simulink model "CLA_Sample"  (R2022b)
settings: Solver=FixedStepAuto  StartTime=0.0  StopTime=Inf  RelTol=1e-3  EnableMultiTasking=on
model workspace (MAT data in the model file):
  ADC_Gain = 1241.21212121
  DAC_Gain = 0.000805860805861
  Inductor_Current_Divider_Gain_Phase_A = 33.4
  Inductor_Current_Divider_Gain_Phase_B = 33.4
  Vbulk_Divider_Gain = 276.854928018
  Vin_Divider_Gain = 556.17352614
undefined symbols (not defined in the file or in its folder): GPTRIP1SEL, GPTRIP2SEL, SCI_A_Transmit, SCI_A_Transmit_Current_Suffix, SCI_A_Transmit_one_shot_Suffix, SCI_A_Transmit_Polarity_Suffix, SCI_A_Transmit_relay_Suffix, SCI_A_Transmit_Vbulk_Suffix, SCI_A_Transmit_Vin_rms_Suffix, SCI_A_Transmit_Vin_Suffix, SCI_A_Transmit_Vmid_Suffix, SCI_A_Transmit_Vp_Suffix, SCI_A_Transmit_Vpfc_Suffix, TZ1, TZ2
libraries: c280xlib x33, simulink x17, c2802xlib x15, c2000lib x1, c2806xlib x1
(part 3 of 5)

== system CLA_Sample/Calibration,RMS, Fault Protection @5kHz/Fault checking/If Action Subsystem ==
  note: Do other fault checks here.
  note: O/P Bulk_UVP-> working but still not perfect.
      | Add more conditons during start up(Not to trigger)
  Action Port : ActionPort  ActionPortLabel=if(u1 ==1)
  Fault Check (Bulk UVP) : Subsystem  Commented=on  TreatAsAtomicUnit=on
  Function-Call Generator : simulink/Ports & Subsystems/Function-Call Generator  sample_time=-1  numberOfIterations=1  DisallowWideOutput=off
  Function-Call Split : FunctionCallSplit  IconShape=distinctive  NumOutputPorts=9  OutputPortLayout=default
  Output Voltage_Latch_OVP : Subsystem  TreatAsAtomicUnit=on
  PFC_en_update_3Phase : Subsystem  TreatAsAtomicUnit=on
  PFC_en_update_Phase_A : Subsystem  TreatAsAtomicUnit=on
  PFC_en_update_Phase_B : Subsystem  TreatAsAtomicUnit=on
  PFC_en_update_Phase_C : Subsystem  TreatAsAtomicUnit=on
  Phase_A_Fault : Subsystem  TreatAsAtomicUnit=on
  Phase_B_Fault : Subsystem  TreatAsAtomicUnit=on
  Phase_C_Fault : Subsystem  TreatAsAtomicUnit=on
  wires:
  Function-Call Generator/1 -> Function-Call Split/1
  Function-Call Split/1 -> Fault Check (Bulk UVP)/Trigger
  Function-Call Split/2 -> Output Voltage_Latch_OVP/Trigger
  Function-Call Split/3 -> Phase_A_Fault/Trigger
  Function-Call Split/4 -> Phase_B_Fault/Trigger
  Function-Call Split/5 -> Phase_C_Fault/Trigger
  Function-Call Split/6 -> PFC_en_update_Phase_A/Trigger
  Function-Call Split/7 -> PFC_en_update_Phase_B/Trigger
  Function-Call Split/8 -> PFC_en_update_Phase_C/Trigger
  Function-Call Split/9 -> PFC_en_update_3Phase/Trigger

== system CLA_Sample/Calibration,RMS, Fault Protection @5kHz/Polarity & Near Zero check/Polarity_Near_zero_Phase_A ==
  note: Unit in Volt
  function : TriggerPort  TriggerType=function-call  VariantControl=(inherit)
  Chart : Stateflow chart  TreatAsAtomicUnit=on
  Constant7 : Constant  Value=0
  Data Store Read2 : DataStoreRead  DataStoreName=Vin_ADC_Average_Phase_A  IndexOptions=Index vector (dialog)  Indices=1  OutputSizes=1
  Data Store Read5 : DataStoreRead  DataStoreName=Vin_1_65_ADC_Phase_A  IndexOptions=Index vector (dialog)  Indices=1  OutputSizes=1
  Data Store Write1 : DataStoreWrite  DataStoreName=Near_Zero_Bar_Phase_A  IndexOptions=Index vector (dialog)  Indices=1  OutputSizes=1
  Data Store Write3 : DataStoreWrite  DataStoreName=Polarity_Phase_A  IndexOptions=Index vector (dialog)  Indices=1  OutputSizes=1
  Near Zero_7V_Analog : Constant  Value=7
  Near_zero : c280xlib/Digital Output  Commented=on  GPIO_Number=GPIO16~GPIO23  GPIO_Bit0=off  GPIO_BIT0_Toggle=off  GPIO_Bit1=off  GPIO_BIT1_Toggle=off  GPIO_Bit2=off  GPIO_BIT2_Toggle=off  GPIO_Bit3=off  GPIO_BIT3_Toggle=off  GPIO_Bit4=off  GPIO_BIT4_Toggle=off  GPIO_Bit5=off  GPIO_BIT5_Toggle=off  GPIO_Bit6=on  GPIO_BIT6_Toggle=off  GPIO_Bit7=off  GPIO_BIT7_Toggle=off
  Polarity : c280xlib/Digital Output  Commented=on  GPIO_Number=GPIO24~GPIO31  GPIO_Bit0=off  GPIO_BIT0_Toggle=off  GPIO_Bit1=on  GPIO_BIT1_Toggle=off  GPIO_Bit2=off  GPIO_BIT2_Toggle=off  GPIO_Bit3=off  GPIO_BIT3_Toggle=off  GPIO_Bit4=off  GPIO_BIT4_Toggle=off  GPIO_Bit5=off  GPIO_BIT5_Toggle=off  GPIO_Bit6=off  GPIO_BIT6_Toggle=off  GPIO_Bit7=off  GPIO_BIT7_Toggle=off
  Subtract2 : Sum  Inputs=+-
  Volt to Number : Subsystem
  wires:
  Constant7/1 -> Chart/2(Vref)
  Volt to Number/1(Out1) -> Chart/3(VZCD_Gap)
  Chart/2(Near_zero) -> Near_zero/1, Data Store Write1/1
  Near Zero_7V_Analog/1 -> Volt to Number/1(In1)
  Chart/1(Polarity) -> Polarity/1, Data Store Write3/1
  Data Store Read5/1 -> Subtract2/2
  Data Store Read2/1 -> Subtract2/1
  Subtract2/1 -> Chart/1(input)

== system CLA_Sample/Calibration,RMS, Fault Protection @5kHz/Polarity & Near Zero check/Polarity_Near_zero_Phase_B ==
  note: Unit in Volt
  function : TriggerPort  TriggerType=function-call  VariantControl=(inherit)
  Chart : Stateflow chart  TreatAsAtomicUnit=on
  Constant7 : Constant  Value=0
  Data Store Read2 : DataStoreRead  DataStoreName=Vin_ADC_Average_Phase_B  IndexOptions=Index vector (dialog)  Indices=1  OutputSizes=1
  Data Store Read5 : DataStoreRead  DataStoreName=Vin_1_65_ADC_Phase_B  IndexOptions=Index vector (dialog)  Indices=1  OutputSizes=1
  Data Store Write1 : DataStoreWrite  DataStoreName=Near_Zero_Bar_Phase_B  IndexOptions=Index vector (dialog)  Indices=1  OutputSizes=1
  Data Store Write3 : DataStoreWrite  DataStoreName=Polarity_Phase_B  IndexOptions=Index vector (dialog)  Indices=1  OutputSizes=1
  Near Zero_7V_Analog : Constant  Value=7
  Near_zero : c280xlib/Digital Output  Commented=on  GPIO_Number=GPIO16~GPIO23  GPIO_Bit0=off  GPIO_BIT0_Toggle=off  GPIO_Bit1=off  GPIO_BIT1_Toggle=off  GPIO_Bit2=off  GPIO_BIT2_Toggle=off  GPIO_Bit3=off  GPIO_BIT3_Toggle=off  GPIO_Bit4=off  GPIO_BIT4_Toggle=off  GPIO_Bit5=off  GPIO_BIT5_Toggle=off  GPIO_Bit6=on  GPIO_BIT6_Toggle=off  GPIO_Bit7=off  GPIO_BIT7_Toggle=off
  Polarity : c280xlib/Digital Output  Commented=on  GPIO_Number=GPIO24~GPIO31  GPIO_Bit0=off  GPIO_BIT0_Toggle=off  GPIO_Bit1=on  GPIO_BIT1_Toggle=off  GPIO_Bit2=off  GPIO_BIT2_Toggle=off  GPIO_Bit3=off  GPIO_BIT3_Toggle=off  GPIO_Bit4=off  GPIO_BIT4_Toggle=off  GPIO_Bit5=off  GPIO_BIT5_Toggle=off  GPIO_Bit6=off  GPIO_BIT6_Toggle=off  GPIO_Bit7=off  GPIO_BIT7_Toggle=off
  Subtract2 : Sum  Inputs=+-
  Volt to Number : Subsystem
  wires:
  Constant7/1 -> Chart/2(Vref)
  Volt to Number/1(Out1) -> Chart/3(VZCD_Gap)
  Chart/2(Near_zero) -> Near_zero/1, Data Store Write1/1
  Near Zero_7V_Analog/1 -> Volt to Number/1(In1)
  Chart/1(Polarity) -> Polarity/1, Data Store Write3/1
  Data Store Read5/1 -> Subtract2/2
  Data Store Read2/1 -> Subtract2/1
  Subtract2/1 -> Chart/1(input)

== system CLA_Sample/Calibration,RMS, Fault Protection @5kHz/Polarity & Near Zero check/Polarity_Near_zero_Phase_C ==
  note: Unit in Volt
  function : TriggerPort  TriggerType=function-call  VariantControl=(inherit)
  Chart : Stateflow chart  TreatAsAtomicUnit=on
  Constant7 : Constant  Value=0
  Data Store Read2 : DataStoreRead  DataStoreName=Vin_ADC_Average_Phase_C  IndexOptions=Index vector (dialog)  Indices=1  OutputSizes=1
  Data Store Read5 : DataStoreRead  DataStoreName=Vin_1_65_ADC_Phase_C  IndexOptions=Index vector (dialog)  Indices=1  OutputSizes=1
  Data Store Write1 : DataStoreWrite  DataStoreName=Near_Zero_Bar_Phase_C  IndexOptions=Index vector (dialog)  Indices=1  OutputSizes=1
  Data Store Write3 : DataStoreWrite  DataStoreName=Polarity_Phase_C  IndexOptions=Index vector (dialog)  Indices=1  OutputSizes=1
  Near Zero_7V_Analog : Constant  Value=7
  Near_zero : c280xlib/Digital Output  Commented=on  GPIO_Number=GPIO16~GPIO23  GPIO_Bit0=off  GPIO_BIT0_Toggle=off  GPIO_Bit1=off  GPIO_BIT1_Toggle=off  GPIO_Bit2=off  GPIO_BIT2_Toggle=off  GPIO_Bit3=off  GPIO_BIT3_Toggle=off  GPIO_Bit4=off  GPIO_BIT4_Toggle=off  GPIO_Bit5=off  GPIO_BIT5_Toggle=off  GPIO_Bit6=on  GPIO_BIT6_Toggle=off  GPIO_Bit7=off  GPIO_BIT7_Toggle=off
  Polarity : c280xlib/Digital Output  Commented=on  GPIO_Number=GPIO24~GPIO31  GPIO_Bit0=off  GPIO_BIT0_Toggle=off  GPIO_Bit1=on  GPIO_BIT1_Toggle=off  GPIO_Bit2=off  GPIO_BIT2_Toggle=off  GPIO_Bit3=off  GPIO_BIT3_Toggle=off  GPIO_Bit4=off  GPIO_BIT4_Toggle=off  GPIO_Bit5=off  GPIO_BIT5_Toggle=off  GPIO_Bit6=off  GPIO_BIT6_Toggle=off  GPIO_Bit7=off  GPIO_BIT7_Toggle=off
  Subtract2 : Sum  Inputs=+-
  Volt to Number : Subsystem
  wires:
  Constant7/1 -> Chart/2(Vref)
  Volt to Number/1(Out1) -> Chart/3(VZCD_Gap)
  Chart/2(Near_zero) -> Near_zero/1, Data Store Write1/1
  Near Zero_7V_Analog/1 -> Volt to Number/1(In1)
  Chart/1(Polarity) -> Polarity/1, Data Store Write3/1
  Data Store Read5/1 -> Subtract2/2
  Data Store Read2/1 -> Subtract2/1
  Subtract2/1 -> Chart/1(input)

== system CLA_Sample/Calibration,RMS, Fault Protection @5kHz/Relay control/ADC Gain ==
  In1 : Inport
  Gain : Gain  Gain=ADC_Gain
  Gain1 : Gain  Gain=1/Vin_Divider_Gain
  Out1 : Outport
  wires:
  Gain1/1 -> Gain/1
  In1/1 -> Gain1/1
  Gain/1 -> Out1/1

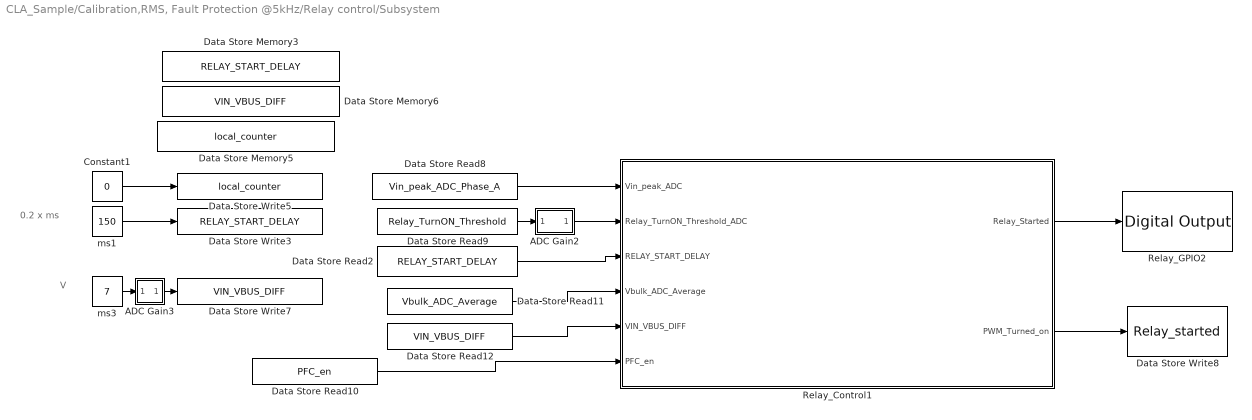
== system CLA_Sample/Calibration,RMS, Fault Protection @5kHz/Relay control/Subsystem ==
  note: 0.2 x ms
  note: V
  ADC Gain2 : Subsystem
  ADC Gain3 : Subsystem
  Constant1 : Constant  Value=0
  Data Store Memory3 : DataStoreMemory  DataStoreName=RELAY_START_DELAY  WriteAfterWriteMsg=warning  ShowAdditionalParam=off
  Data Store Memory5 : DataStoreMemory  DataStoreName=local_counter  WriteAfterWriteMsg=warning  ShowAdditionalParam=off
  Data Store Memory6 : DataStoreMemory  DataStoreName=VIN_VBUS_DIFF  WriteAfterWriteMsg=warning  ShowAdditionalParam=off
  Data Store Read10 : DataStoreRead  DataStoreName=PFC_en  IndexOptions=Index vector (dialog)  Indices=1  OutputSizes=1
  Data Store Read11 : DataStoreRead  DataStoreName=Vbulk_ADC_Average  IndexOptions=Index vector (dialog)  Indices=1  OutputSizes=1
  Data Store Read12 : DataStoreRead  DataStoreName=VIN_VBUS_DIFF  IndexOptions=Index vector (dialog)  Indices=1  OutputSizes=1
  Data Store Read2 : DataStoreRead  DataStoreName=RELAY_START_DELAY  IndexOptions=Index vector (dialog)  Indices=1  OutputSizes=1
  Data Store Read8 : DataStoreRead  DataStoreName=Vin_peak_ADC_Phase_A  IndexOptions=Index vector (dialog)  Indices=1  OutputSizes=1
  Data Store Read9 : DataStoreRead  DataStoreName=Relay_TurnON_Threshold  IndexOptions=Index vector (dialog)  Indices=1  OutputSizes=1
  Data Store Write3 : DataStoreWrite  DataStoreName=RELAY_START_DELAY  IndexOptions=Index vector (dialog)  Indices=1  OutputSizes=1
  Data Store Write5 : DataStoreWrite  DataStoreName=local_counter  IndexOptions=Index vector (dialog)  Indices=1  OutputSizes=1
  Data Store Write7 : DataStoreWrite  DataStoreName=VIN_VBUS_DIFF  IndexOptions=Index vector (dialog)  Indices=1  OutputSizes=1
  Data Store Write8 : DataStoreWrite  DataStoreName=Relay_started  IndexOptions=Index vector (dialog)  Indices=1  OutputSizes=1
  Relay_Control1 : Stateflow chart  TreatAsAtomicUnit=on
  Relay_GPIO2 : c280xlib/Digital Output  GPIO_Number=GPIO8~GPIO15  GPIO_Bit0=on  GPIO_BIT0_Toggle=off  GPIO_Bit1=off  GPIO_BIT1_Toggle=off  GPIO_Bit2=off  GPIO_BIT2_Toggle=off  GPIO_Bit3=off  GPIO_BIT3_Toggle=off  GPIO_Bit4=off  GPIO_BIT4_Toggle=off  GPIO_Bit5=off  GPIO_BIT5_Toggle=off  GPIO_Bit6=off  GPIO_BIT6_Toggle=off  GPIO_Bit7=off  GPIO_BIT7_Toggle=off
  ms1 : Constant  Value=150
  ms3 : Constant  Value=7
  wires:
  Data Store Read8/1 -> Relay_Control1/1(Vin_peak_ADC)
  Data Store Read11/1 -> Relay_Control1/4(Vbulk_ADC_Average)
  Relay_Control1/2(PWM_Turned_on) -> Data Store Write8/1
  Data Store Read9/1 -> ADC Gain2/1(In1)
  Data Store Read2/1 -> Relay_Control1/3(RELAY_START_DELAY)
  Data Store Read10/1 -> Relay_Control1/6(PFC_en)
  ADC Gain3/1(Out1) -> Data Store Write7/1
  ms1/1 -> Data Store Write3/1
  ms3/1 -> ADC Gain3/1(In1)
  Relay_Control1/1(Relay_Started) -> Relay_GPIO2/1
  ADC Gain2/1(Out1) -> Relay_Control1/2(Relay_TurnON_Threshold_ADC)
  Constant1/1 -> Data Store Write5/1
  Data Store Read12/1 -> Relay_Control1/5(VIN_VBUS_DIFF)

== system CLA_Sample/Calibration,RMS, Fault Protection @5kHz/Voltage RMS//Averag Calculation/Phase_A ==
  function : TriggerPort  TriggerType=function-call  VariantControl=(inherit)
  Function-Call Generator : simulink/Ports & Subsystems/Function-Call Generator  sample_time=-1  numberOfIterations=1  DisallowWideOutput=off
  Function-Call Split : FunctionCallSplit  IconShape=distinctive  NumOutputPorts=3  OutputPortLayout=default
  RMS Current Calculation_Phase_A : Subsystem  TreatAsAtomicUnit=on
  RMS Voltage Calculation_Phase_A : Subsystem  TreatAsAtomicUnit=on
  Vin_ADC Averaging_Phase_A : Subsystem  TreatAsAtomicUnit=on
  wires:
  Function-Call Generator/1 -> Function-Call Split/1
  Function-Call Split/1 -> RMS Voltage Calculation_Phase_A/Trigger
  Function-Call Split/2 -> RMS Current Calculation_Phase_A/Trigger
  Function-Call Split/3 -> Vin_ADC Averaging_Phase_A/Trigger

== system CLA_Sample/Calibration,RMS, Fault Protection @5kHz/Voltage RMS//Averag Calculation/Phase_B ==
  function : TriggerPort  TriggerType=function-call  VariantControl=(inherit)
  Function-Call Generator : simulink/Ports & Subsystems/Function-Call Generator  sample_time=-1  numberOfIterations=1  DisallowWideOutput=off
  Function-Call Split : FunctionCallSplit  IconShape=distinctive  NumOutputPorts=3  OutputPortLayout=default
  RMS Current Calculation_Phase_B : Subsystem  TreatAsAtomicUnit=on
  RMS Voltage Calculation_Phase_B : Subsystem  TreatAsAtomicUnit=on
  Vin_ADC Averaging_Phase_B : Subsystem  TreatAsAtomicUnit=on
  wires:
  Function-Call Generator/1 -> Function-Call Split/1
  Function-Call Split/1 -> RMS Voltage Calculation_Phase_B/Trigger
  Function-Call Split/2 -> RMS Current Calculation_Phase_B/Trigger
  Function-Call Split/3 -> Vin_ADC Averaging_Phase_B/Trigger

== system CLA_Sample/Calibration,RMS, Fault Protection @5kHz/Voltage RMS//Averag Calculation/Phase_C ==
  function : TriggerPort  TriggerType=function-call  VariantControl=(inherit)
  Function-Call Generator : simulink/Ports & Subsystems/Function-Call Generator  sample_time=-1  numberOfIterations=1  DisallowWideOutput=off
  Function-Call Split : FunctionCallSplit  IconShape=distinctive  NumOutputPorts=3  OutputPortLayout=default
  RMS Current Calculation_Phase_C : Subsystem  TreatAsAtomicUnit=on
  RMS Voltage Calculation_Phase_C : Subsystem  TreatAsAtomicUnit=on
  Vin_ADC Averaging_Phase_C : Subsystem  TreatAsAtomicUnit=on
  wires:
  Function-Call Generator/1 -> Function-Call Split/1
  Function-Call Split/1 -> RMS Voltage Calculation_Phase_C/Trigger
  Function-Call Split/2 -> RMS Current Calculation_Phase_C/Trigger
  Function-Call Split/3 -> Vin_ADC Averaging_Phase_C/Trigger

== system CLA_Sample/Calibration,RMS, Fault Protection @5kHz/Voltage RMS//Averag Calculation/Vbulk_ADC Averaging ==
  note: Low pass filter :
      | 1kHz bandwidth with 5kHz switching freq
  function : TriggerPort  TriggerType=function-call  VariantControl=(inherit)
  Chart1 : Stateflow chart  TreatAsAtomicUnit=on
  Constant1 : Constant  Value=0.38586954
  Constant2 : Constant  Value=0.38586954
  Constant3 : Constant  Value=-0.22826091
  Data Store Read1 : DataStoreRead  DataStoreName=Vbulk_ADC  IndexOptions=Index vector (dialog)  Indices=1  OutputSizes=1
  Vout_ADC_Average : DataStoreWrite  DataStoreName=Vbulk_ADC_Average  IndexOptions=Index vector (dialog)  Indices=1  OutputSizes=1
  wires:
  Chart1/1(output_y) -> Vout_ADC_Average/1
  Data Store Read1/1 -> Chart1/1(input_u)
  [b0] -> Chart1/2(b0)
  [b1] -> Chart1/3(b1)
  [a1] -> Chart1/4(a1)
  Constant2/1 -> [b1]
  Constant1/1 -> [b0]
  Constant3/1 -> [a1]

== system CLA_Sample/PWM Update @65KHz/Closed loop PWM generation (Control)/If Action Subsystem ==
  Action Port : ActionPort  ActionPortLabel=if((u1 ==1) & (u2==1))
  CLA Task : c2806xlib/CLA Task  taskNumber=1  intSource=Software  wait=off  sampleTime=0.2  claType=0  softTrigSelected=1  enableInterrupt=on
  Function-Call Subsystem : Subsystem  TreatAsAtomicUnit=on
  wires:
  CLA Task/1 -> Function-Call Subsystem/Trigger

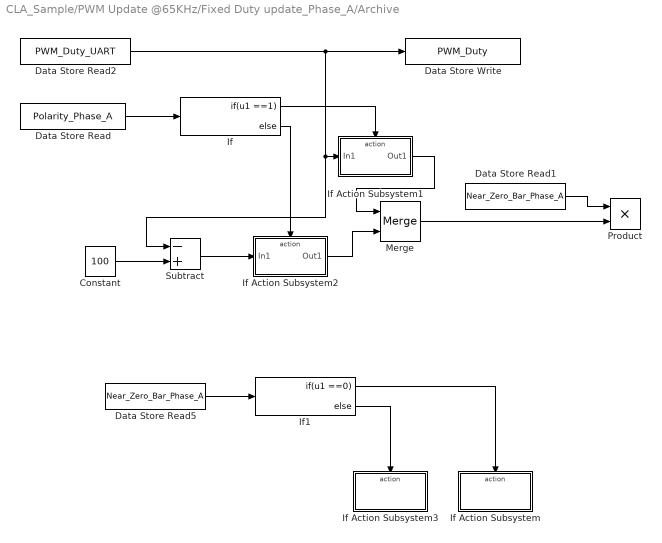
== system CLA_Sample/PWM Update @65KHz/Fixed Duty update_Phase_A/Archive ==
  Constant : Constant  Value=100
  Data Store Read : DataStoreRead  DataStoreName=Polarity_Phase_A  IndexOptions=Index vector (dialog)  Indices=1  OutputSizes=1
  Data Store Read1 : DataStoreRead  DataStoreName=Near_Zero_Bar_Phase_A  IndexOptions=Index vector (dialog)  Indices=1  OutputSizes=1
  Data Store Read2 : DataStoreRead  DataStoreName=PWM_Duty_UART  IndexOptions=Index vector (dialog)  Indices=1  OutputSizes=1
  Data Store Read5 : DataStoreRead  DataStoreName=Near_Zero_Bar_Phase_A  IndexOptions=Index vector (dialog)  Indices=1  OutputSizes=1
  Data Store Write : DataStoreWrite  DataStoreName=PWM_Duty  IndexOptions=Index vector (dialog)  Indices=1  OutputSizes=1
  If : If  IfExpression=u1 ==1
  If Action Subsystem : Subsystem  TreatAsAtomicUnit=on
  If Action Subsystem1 : Subsystem  TreatAsAtomicUnit=on
  If Action Subsystem2 : Subsystem  TreatAsAtomicUnit=on
  If Action Subsystem3 : Subsystem  TreatAsAtomicUnit=on
  If1 : If  IfExpression=u1 ==0
  Merge : Merge
  Product : Product
  Subtract : Sum  Inputs=-+
  wires:
  If/1 -> If Action Subsystem1/Action
  Data Store Read2/1 -> If Action Subsystem1/1(In1), Subtract/1, Data Store Write/1
  Merge/1 -> Product/2
  If Action Subsystem2/1(Out1) -> Merge/2
  Constant/1 -> Subtract/2
  Data Store Read/1 -> If/1
  Subtract/1 -> If Action Subsystem2/1(In1)
  Data Store Read1/1 -> Product/1
  If/2 -> If Action Subsystem2/Action
  If Action Subsystem1/1(Out1) -> Merge/1
  If1/1 -> If Action Subsystem/Action
  Data Store Read5/1 -> If1/1
  If1/2 -> If Action Subsystem3/Action

== system CLA_Sample/PWM Update @65KHz/Fixed Duty update_Phase_A/If Action Subsystem3 ==
  Action Port : ActionPort  ActionPortLabel=if(u1==1 & u2==0)
  Constant : Constant
  Digital Output : c280xlib/Digital Output  GPIO_Number=GPIO16~GPIO23  GPIO_Bit0=off  GPIO_BIT0_Toggle=off  GPIO_Bit1=off  GPIO_BIT1_Toggle=off  GPIO_Bit2=off  GPIO_BIT2_Toggle=off  GPIO_Bit3=off  GPIO_BIT3_Toggle=off  GPIO_Bit4=off  GPIO_BIT4_Toggle=off  GPIO_Bit5=off  GPIO_BIT5_Toggle=off  GPIO_Bit6=on  GPIO_BIT6_Toggle=off  GPIO_Bit7=off  GPIO_BIT7_Toggle=off
  wires:
  Constant/1 -> Digital Output/1

== system CLA_Sample/PWM Update @65KHz/Fixed Duty update_Phase_A/If Action Subsystem4 ==
  Action Port : ActionPort  ActionPortLabel=elseif(u1==1 & u2==1)
  Constant : Constant  Value=0
  Digital Output : c280xlib/Digital Output  GPIO_Number=GPIO16~GPIO23  GPIO_Bit0=off  GPIO_BIT0_Toggle=off  GPIO_Bit1=off  GPIO_BIT1_Toggle=off  GPIO_Bit2=off  GPIO_BIT2_Toggle=off  GPIO_Bit3=off  GPIO_BIT3_Toggle=off  GPIO_Bit4=off  GPIO_BIT4_Toggle=off  GPIO_Bit5=off  GPIO_BIT5_Toggle=off  GPIO_Bit6=on  GPIO_BIT6_Toggle=off  GPIO_Bit7=off  GPIO_BIT7_Toggle=off
  wires:
  Constant/1 -> Digital Output/1

== system CLA_Sample/PWM Update @65KHz/Fixed Duty update_Phase_A/Subsystem1 ==
  Frequency(kHz) : Inport
  Duty(%) : Inport  Port=2
  Constant1 : Constant  Value=90E6
  Divide : Product  Inputs=*/  RndMeth=Zero  SaturateOnIntegerOverflow=on
  Gain : Gain  Gain=1000
  Gain1 : Gain  Gain=1/100
  Gain2 : Gain  Gain=0.5
  Product1 : Product
  Out1 : Outport
  Out2 : Outport  Port=2
  Out3 : Outport  Port=3
  wires:
  Gain2/1 -> Out3/1
  Gain1/1 -> Product1/2
  Product1/1 -> Gain2/1, Out2/1
  Duty(%)/1 -> Gain1/1
  Divide/1 -> Out1/1, Product1/1
  Gain/1 -> Divide/2
  Constant1/1 -> Divide/1
  Frequency(kHz)/1 -> Gain/1

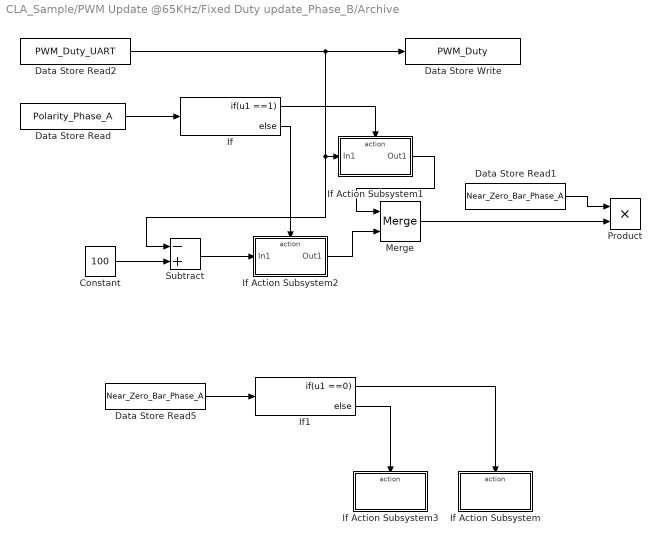
== system CLA_Sample/PWM Update @65KHz/Fixed Duty update_Phase_B/Archive ==
  Constant : Constant  Value=100
  Data Store Read : DataStoreRead  DataStoreName=Polarity_Phase_A  IndexOptions=Index vector (dialog)  Indices=1  OutputSizes=1
  Data Store Read1 : DataStoreRead  DataStoreName=Near_Zero_Bar_Phase_A  IndexOptions=Index vector (dialog)  Indices=1  OutputSizes=1
  Data Store Read2 : DataStoreRead  DataStoreName=PWM_Duty_UART  IndexOptions=Index vector (dialog)  Indices=1  OutputSizes=1
  Data Store Read5 : DataStoreRead  DataStoreName=Near_Zero_Bar_Phase_A  IndexOptions=Index vector (dialog)  Indices=1  OutputSizes=1
  Data Store Write : DataStoreWrite  DataStoreName=PWM_Duty  IndexOptions=Index vector (dialog)  Indices=1  OutputSizes=1
  If : If  IfExpression=u1 ==1
  If Action Subsystem : Subsystem  TreatAsAtomicUnit=on
  If Action Subsystem1 : Subsystem  TreatAsAtomicUnit=on
  If Action Subsystem2 : Subsystem  TreatAsAtomicUnit=on
  If Action Subsystem3 : Subsystem  TreatAsAtomicUnit=on
  If1 : If  IfExpression=u1 ==0
  Merge : Merge
  Product : Product
  Subtract : Sum  Inputs=-+
  wires:
  If/1 -> If Action Subsystem1/Action
  Data Store Read2/1 -> If Action Subsystem1/1(In1), Subtract/1, Data Store Write/1
  Merge/1 -> Product/2
  If Action Subsystem2/1(Out1) -> Merge/2
  Constant/1 -> Subtract/2
  Data Store Read/1 -> If/1
  Subtract/1 -> If Action Subsystem2/1(In1)
  Data Store Read1/1 -> Product/1
  If/2 -> If Action Subsystem2/Action
  If Action Subsystem1/1(Out1) -> Merge/1
  If1/1 -> If Action Subsystem/Action
  Data Store Read5/1 -> If1/1
  If1/2 -> If Action Subsystem3/Action

== system CLA_Sample/PWM Update @65KHz/Fixed Duty update_Phase_B/Subsystem1 ==
  Frequency(kHz) : Inport
  Duty(%) : Inport  Port=2
  Constant1 : Constant  Value=90E6
  Divide : Product  Inputs=*/  RndMeth=Zero  SaturateOnIntegerOverflow=on
  Gain : Gain  Gain=1000
  Gain1 : Gain  Gain=1/100
  Gain2 : Gain  Gain=0.5
  Product1 : Product
  Out1 : Outport
  Out2 : Outport  Port=2
  Out3 : Outport  Port=3
  wires:
  Gain2/1 -> Out3/1
  Gain1/1 -> Product1/2
  Product1/1 -> Gain2/1, Out2/1
  Duty(%)/1 -> Gain1/1
  Divide/1 -> Out1/1, Product1/1
  Gain/1 -> Divide/2
  Constant1/1 -> Divide/1
  Frequency(kHz)/1 -> Gain/1

== system CLA_Sample/PWM Update @65KHz/Fixed Duty update_Phase_C/Archive ==
  Constant : Constant  Value=100
  Data Store Read : DataStoreRead  DataStoreName=Polarity_Phase_A  IndexOptions=Index vector (dialog)  Indices=1  OutputSizes=1
  Data Store Read1 : DataStoreRead  DataStoreName=Near_Zero_Bar_Phase_A  IndexOptions=Index vector (dialog)  Indices=1  OutputSizes=1
  Data Store Read2 : DataStoreRead  DataStoreName=PWM_Duty_UART  IndexOptions=Index vector (dialog)  Indices=1  OutputSizes=1
  Data Store Read5 : DataStoreRead  DataStoreName=Near_Zero_Bar_Phase_A  IndexOptions=Index vector (dialog)  Indices=1  OutputSizes=1
  Data Store Write : DataStoreWrite  DataStoreName=PWM_Duty  IndexOptions=Index vector (dialog)  Indices=1  OutputSizes=1
  If : If  IfExpression=u1 ==1
  If Action Subsystem : Subsystem  TreatAsAtomicUnit=on
  If Action Subsystem1 : Subsystem  TreatAsAtomicUnit=on
  If Action Subsystem2 : Subsystem  TreatAsAtomicUnit=on
  If Action Subsystem3 : Subsystem  TreatAsAtomicUnit=on
  If1 : If  IfExpression=u1 ==0
  Merge : Merge
  Product : Product
  Subtract : Sum  Inputs=-+
  wires:
  If/1 -> If Action Subsystem1/Action
  Data Store Read2/1 -> If Action Subsystem1/1(In1), Subtract/1, Data Store Write/1
  Merge/1 -> Product/2
  If Action Subsystem2/1(Out1) -> Merge/2
  Constant/1 -> Subtract/2
  Data Store Read/1 -> If/1
  Subtract/1 -> If Action Subsystem2/1(In1)
  Data Store Read1/1 -> Product/1
  If/2 -> If Action Subsystem2/Action
  If Action Subsystem1/1(Out1) -> Merge/1
  If1/1 -> If Action Subsystem/Action
  Data Store Read5/1 -> If1/1
  If1/2 -> If Action Subsystem3/Action

== system CLA_Sample/PWM Update @65KHz/Fixed Duty update_Phase_C/Subsystem1 ==
  Frequency(kHz) : Inport
  Duty(%) : Inport  Port=2
  Constant1 : Constant  Value=90E6
  Divide : Product  Inputs=*/  RndMeth=Zero  SaturateOnIntegerOverflow=on
  Gain : Gain  Gain=1000
  Gain1 : Gain  Gain=1/100
  Gain2 : Gain  Gain=0.5
  Product1 : Product
  Out1 : Outport
  Out2 : Outport  Port=2
  Out3 : Outport  Port=3
  wires:
  Gain2/1 -> Out3/1
  Gain1/1 -> Product1/2
  Product1/1 -> Gain2/1, Out2/1
  Duty(%)/1 -> Gain1/1
  Divide/1 -> Out1/1, Product1/1
  Gain/1 -> Divide/2
  Constant1/1 -> Divide/1
  Frequency(kHz)/1 -> Gain/1

== system CLA_Sample/UART reporting @ 1Hz/Data_calculation/DataCalculation_Phase_A ==
  function : TriggerPort  TriggerType=function-call  VariantControl=(inherit)
  Data Store Read : DataStoreRead  DataStoreName=Inductor_Current_ADC_Phase_A  IndexOptions=Index vector (dialog)  Indices=1  OutputSizes=1
  Data Store Read1 : DataStoreRead  DataStoreName=Vin_ADC_Average_Phase_A  IndexOptions=Index vector (dialog)  Indices=1  OutputSizes=1
  Data Store Read3 : DataStoreRead  DataStoreName=Inductor_Current_1_65_ADC_Phase_A  IndexOptions=Index vector (dialog)  Indices=1  OutputSizes=1
  Data Store Read4 : DataStoreRead  DataStoreName=Vin_1_65_ADC_Phase_A  IndexOptions=Index vector (dialog)  Indices=1  OutputSizes=1
  Data Store Write2 : DataStoreWrite  DataStoreName=Inductor_Current_Phase_A  IndexOptions=Index vector (dialog)  Indices=1  OutputSizes=1
  Data Store Write4 : DataStoreWrite  DataStoreName=Vin_Phase_A  IndexOptions=Index vector (dialog)  Indices=1  OutputSizes=1
  Gain2 : Gain  Gain=DAC_Gain
  Gain3 : Gain  Gain=Inductor_Current_Divider_Gain_Phase_A
  Gain4 : Gain  Gain=DAC_Gain
  Gain5 : Gain  Gain=Vin_Divider_Gain
  Gain6 : Gain  Gain=100
  Subtract1 : Sum  Inputs=+-
  Subtract2 : Sum  Inputs=+-
  wires:
  Gain5/1 -> Data Store Write4/1
  Subtract2/1 -> Gain2/1
  Gain4/1 -> Gain5/1
  Subtract1/1 -> Gain4/1
  Gain6/1 -> Data Store Write2/1
  Data Store Read4/1 -> Subtract1/2
  Gain3/1 -> Gain6/1
  Data Store Read3/1 -> Subtract2/2
  Data Store Read1/1 -> Subtract1/1
  Gain2/1 -> Gain3/1
  Data Store Read/1 -> Subtract2/1

== system CLA_Sample/UART reporting @ 1Hz/Data_calculation/DataCalculation_Phase_B ==
  function : TriggerPort  TriggerType=function-call  VariantControl=(inherit)
  Data Store Read : DataStoreRead  DataStoreName=Inductor_Current_ADC_Phase_B  IndexOptions=Index vector (dialog)  Indices=1  OutputSizes=1
  Data Store Read1 : DataStoreRead  DataStoreName=Vin_ADC_Average_Phase_B  IndexOptions=Index vector (dialog)  Indices=1  OutputSizes=1
  Data Store Read3 : DataStoreRead  DataStoreName=Inductor_Current_1_65_ADC_Phase_B  IndexOptions=Index vector (dialog)  Indices=1  OutputSizes=1
  Data Store Read4 : DataStoreRead  DataStoreName=Vin_1_65_ADC_Phase_B  IndexOptions=Index vector (dialog)  Indices=1  OutputSizes=1
  Data Store Write2 : DataStoreWrite  DataStoreName=Inductor_Current_Phase_B  IndexOptions=Index vector (dialog)  Indices=1  OutputSizes=1
  Data Store Write4 : DataStoreWrite  DataStoreName=Vin_Phase_B  IndexOptions=Index vector (dialog)  Indices=1  OutputSizes=1
  Gain2 : Gain  Gain=DAC_Gain
  Gain3 : Gain  Gain=Inductor_Current_Divider_Gain_Phase_B
  Gain4 : Gain  Gain=DAC_Gain
  Gain5 : Gain  Gain=Vin_Divider_Gain
  Gain6 : Gain  Gain=100
  Subtract1 : Sum  Inputs=+-
  Subtract2 : Sum  Inputs=+-
  wires:
  Gain5/1 -> Data Store Write4/1
  Subtract2/1 -> Gain2/1
  Gain4/1 -> Gain5/1
  Subtract1/1 -> Gain4/1
  Gain6/1 -> Data Store Write2/1
  Data Store Read4/1 -> Subtract1/2
  Gain3/1 -> Gain6/1
  Data Store Read3/1 -> Subtract2/2
  Data Store Read1/1 -> Subtract1/1
  Gain2/1 -> Gain3/1
  Data Store Read/1 -> Subtract2/1

== system CLA_Sample/UART reporting @ 1Hz/Data_calculation/DataCalculation_Phase_C ==
  function : TriggerPort  TriggerType=function-call  VariantControl=(inherit)
  Data Store Read : DataStoreRead  DataStoreName=Inductor_Current_ADC_Phase_C  IndexOptions=Index vector (dialog)  Indices=1  OutputSizes=1
  Data Store Read1 : DataStoreRead  DataStoreName=Vin_ADC_Average_Phase_C  IndexOptions=Index vector (dialog)  Indices=1  OutputSizes=1
  Data Store Read3 : DataStoreRead  DataStoreName=Inductor_Current_1_65_ADC_Phase_C  IndexOptions=Index vector (dialog)  Indices=1  OutputSizes=1
  Data Store Read4 : DataStoreRead  DataStoreName=Vin_1_65_ADC_Phase_C  IndexOptions=Index vector (dialog)  Indices=1  OutputSizes=1
  Data Store Write2 : DataStoreWrite  DataStoreName=Inductor_Current_Phase_C  IndexOptions=Index vector (dialog)  Indices=1  OutputSizes=1
  Data Store Write4 : DataStoreWrite  DataStoreName=Vin_Phase_C  IndexOptions=Index vector (dialog)  Indices=1  OutputSizes=1
  Gain2 : Gain  Gain=DAC_Gain
  Gain3 : Gain  Gain=Inductor_Current_Divider_Gain_Phase_B
  Gain4 : Gain  Gain=DAC_Gain
  Gain5 : Gain  Gain=Vin_Divider_Gain
  Gain6 : Gain  Gain=100
  Subtract1 : Sum  Inputs=+-
  Subtract2 : Sum  Inputs=+-
  wires:
  Gain5/1 -> Data Store Write4/1
  Subtract2/1 -> Gain2/1
  Gain4/1 -> Gain5/1
  Subtract1/1 -> Gain4/1
  Gain6/1 -> Data Store Write2/1
  Data Store Read4/1 -> Subtract1/2
  Gain3/1 -> Gain6/1
  Data Store Read3/1 -> Subtract2/2
  Data Store Read1/1 -> Subtract1/1
  Gain2/1 -> Gain3/1
  Data Store Read/1 -> Subtract2/1

== system CLA_Sample/UART reporting @ 1Hz/Data_calculation/Vbulk&Vmid ==
  function : TriggerPort  TriggerType=function-call  VariantControl=(inherit)
  Data Store Read1 : DataStoreRead  DataStoreName=Vmid_ADC  IndexOptions=Index vector (dialog)  Indices=1  OutputSizes=1
  Data Store Read2 : DataStoreRead  DataStoreName=Vbulk_ADC_Average  IndexOptions=Index vector (dialog)  Indices=1  OutputSizes=1
  Data Store Write1 : DataStoreWrite  DataStoreName=Vbulk  IndexOptions=Index vector (dialog)  Indices=1  OutputSizes=1
  Data Store Write2 : DataStoreWrite  DataStoreName=Vmid  IndexOptions=Index vector (dialog)  Indices=1  OutputSizes=1
  Gain1 : Gain  Gain=DAC_Gain
  Gain2 : Gain  Gain=DAC_Gain
  Gain3 : Gain  Gain=155.47
  Gain7 : Gain  Gain=Vbulk_Divider_Gain  OutDataTypeStr=double
  wires:
  Gain7/1 -> Data Store Write1/1
  Gain1/1 -> Gain7/1
  Data Store Read2/1 -> Gain1/1
  Gain3/1 -> Data Store Write2/1
  Gain2/1 -> Gain3/1
  Data Store Read1/1 -> Gain2/1

== system CLA_Sample/UART reporting @ 1Hz/Phase_A/Duty_control_loop_Phase_A ==
  function : TriggerPort  TriggerType=function-call  VariantControl=(inherit)
  Data Store Read : DataStoreRead  Commented=on  DataStoreName=Vbulk_ADC_Average  IndexOptions=Index vector (dialog)  Indices=1  OutputSizes=1
  Data Store Read1 : DataStoreRead  DataStoreName=ePWM2A_CMPA_Phase_A  IndexOptions=Index vector (dialog)  Indices=1  OutputSizes=1
  Function Caller1 : FunctionCaller  FunctionPrototype=SCI_A_Transmit(u)  InputArgumentSpecifications=<Enter example>  OutputArgumentSpecifications=<Enter example>
  Function Caller2 : FunctionCaller  FunctionPrototype=SCI_A_Transmit_Polarity_Suffix()  InputArgumentSpecifications=<Enter example>  OutputArgumentSpecifications=<Enter example>
  Gain1 : Gain  Commented=on  Gain=DAC_Gain
  Gain7 : Gain  Commented=on  Gain=Vbulk_Divider_Gain
  wires:
  Data Store Read/1 -> Gain1/1
  Gain1/1 -> Gain7/1
  Data Store Read1/1 -> Function Caller1/1

== system CLA_Sample/UART reporting @ 1Hz/Phase_A/Send Inductor_Current (A) ==
  function : TriggerPort  TriggerType=function-call  VariantControl=(inherit)
  Data Store Read : DataStoreRead  DataStoreName=Iin_rms_Phase_A  IndexOptions=Index vector (dialog)  Indices=1  OutputSizes=1
  Function Caller1 : FunctionCaller  FunctionPrototype=SCI_A_Transmit(u)  InputArgumentSpecifications=<Enter example>  OutputArgumentSpecifications=<Enter example>
  Function Caller2 : FunctionCaller  FunctionPrototype=SCI_A_Transmit_Current_Suffix()  InputArgumentSpecifications=<Enter example>  OutputArgumentSpecifications=<Enter example>
  wires:
  Data Store Read/1 -> Function Caller1/1

== system CLA_Sample/UART reporting @ 1Hz/Phase_A/Send PFC_en_Phase_A ==
  function : TriggerPort  TriggerType=function-call  VariantControl=(inherit)
  Data Store Read : DataStoreRead  DataStoreName=PFC_en_Phase_A  IndexOptions=Index vector (dialog)  Indices=1  OutputSizes=1
  Function Caller1 : FunctionCaller  FunctionPrototype=SCI_A_Transmit(u)  InputArgumentSpecifications=<Enter example>  OutputArgumentSpecifications=<Enter example>
  Function Caller2 : FunctionCaller  FunctionPrototype=SCI_A_Transmit_Vp_Suffix()  InputArgumentSpecifications=<Enter example>  OutputArgumentSpecifications=<Enter example>
  wires:
  Data Store Read/1 -> Function Caller1/1

== system CLA_Sample/UART reporting @ 1Hz/Phase_A/Send Vin (V) ==
  function : TriggerPort  TriggerType=function-call  VariantControl=(inherit)
  Data Store Read1 : DataStoreRead  DataStoreName=Vin_Phase_A  IndexOptions=Index vector (dialog)  Indices=1  OutputSizes=1
  Function Caller1 : FunctionCaller  FunctionPrototype=SCI_A_Transmit(u)  InputArgumentSpecifications=<Enter example>  OutputArgumentSpecifications=<Enter example>
  Function Caller2 : FunctionCaller  FunctionPrototype=SCI_A_Transmit_Vin_Suffix()  InputArgumentSpecifications=<Enter example>  OutputArgumentSpecifications=<Enter example>
  wires:
  Data Store Read1/1 -> Function Caller1/1

== system CLA_Sample/UART reporting @ 1Hz/Phase_A/Send Vin_rms (V) ==
  function : TriggerPort  TriggerType=function-call  VariantControl=(inherit)
  Data Store Read1 : DataStoreRead  DataStoreName=Vin_rms_Phase_A  IndexOptions=Index vector (dialog)  Indices=1  OutputSizes=1
  Function Caller1 : FunctionCaller  FunctionPrototype=SCI_A_Transmit(u)  InputArgumentSpecifications=<Enter example>  OutputArgumentSpecifications=<Enter example>
  Function Caller2 : FunctionCaller  FunctionPrototype=SCI_A_Transmit_Vin_rms_Suffix()  InputArgumentSpecifications=<Enter example>  OutputArgumentSpecifications=<Enter example>
  wires:
  Data Store Read1/1 -> Function Caller1/1

== system CLA_Sample/UART reporting @ 1Hz/Phase_B/Duty_control_loop_Phase_B ==
  function : TriggerPort  TriggerType=function-call  VariantControl=(inherit)
  Data Store Read : DataStoreRead  Commented=on  DataStoreName=Vbulk_ADC_Average  IndexOptions=Index vector (dialog)  Indices=1  OutputSizes=1
  Data Store Read1 : DataStoreRead  DataStoreName=ePWM1A_CMPA_Phase_B  IndexOptions=Index vector (dialog)  Indices=1  OutputSizes=1
  Function Caller1 : FunctionCaller  FunctionPrototype=SCI_A_Transmit(u)  InputArgumentSpecifications=<Enter example>  OutputArgumentSpecifications=<Enter example>
  Function Caller2 : FunctionCaller  FunctionPrototype=SCI_A_Transmit_Polarity_Suffix()  InputArgumentSpecifications=<Enter example>  OutputArgumentSpecifications=<Enter example>
  Gain1 : Gain  Commented=on  Gain=DAC_Gain
  Gain7 : Gain  Commented=on  Gain=Vbulk_Divider_Gain
  Phase_B : Constant  Commented=on  Value=[66]  OutDataTypeStr=uint8
  SCI Transmit : c280xlib/SCI Transmit  Commented=on  sciModule=A  dataHead=''  dataTail=10  blockingMode=on  outputStatus=off
  wires:
  Data Store Read/1 -> Gain1/1
  Gain1/1 -> Gain7/1
  Data Store Read1/1 -> Function Caller1/1
  Phase_B/1 -> SCI Transmit/1

== system CLA_Sample/UART reporting @ 1Hz/Phase_B/Send Inductor_Current (A) ==
  function : TriggerPort  TriggerType=function-call  VariantControl=(inherit)
  Data Store Read : DataStoreRead  DataStoreName=Iin_rms_Phase_B  IndexOptions=Index vector (dialog)  Indices=1  OutputSizes=1
  Function Caller1 : FunctionCaller  FunctionPrototype=SCI_A_Transmit(u)  InputArgumentSpecifications=<Enter example>  OutputArgumentSpecifications=<Enter example>
  Function Caller2 : FunctionCaller  FunctionPrototype=SCI_A_Transmit_Current_Suffix()  InputArgumentSpecifications=<Enter example>  OutputArgumentSpecifications=<Enter example>
  Phase_B : Constant  Commented=on  Value=[66]  OutDataTypeStr=uint8
  SCI Transmit : c280xlib/SCI Transmit  Commented=on  sciModule=A  dataHead=''  dataTail=10  blockingMode=on  outputStatus=off
  wires:
  Data Store Read/1 -> Function Caller1/1
  Phase_B/1 -> SCI Transmit/1

== system CLA_Sample/UART reporting @ 1Hz/Phase_B/Send PFC_en_Phase_B ==
  function : TriggerPort  TriggerType=function-call  VariantControl=(inherit)
  Data Store Read : DataStoreRead  DataStoreName=PFC_en_Phase_B  IndexOptions=Index vector (dialog)  Indices=1  OutputSizes=1
  Function Caller1 : FunctionCaller  FunctionPrototype=SCI_A_Transmit(u)  InputArgumentSpecifications=<Enter example>  OutputArgumentSpecifications=<Enter example>
  Function Caller2 : FunctionCaller  FunctionPrototype=SCI_A_Transmit_Vp_Suffix()  InputArgumentSpecifications=<Enter example>  OutputArgumentSpecifications=<Enter example>
  Phase_B : Constant  Commented=on  Value=[66]  OutDataTypeStr=uint8
  SCI Transmit : c280xlib/SCI Transmit  Commented=on  sciModule=A  dataHead=''  dataTail=10  blockingMode=on  outputStatus=off
  wires:
  Data Store Read/1 -> Function Caller1/1
  Phase_B/1 -> SCI Transmit/1

== system CLA_Sample/UART reporting @ 1Hz/Phase_B/Send Vin (V) ==
  function : TriggerPort  TriggerType=function-call  VariantControl=(inherit)
  Data Store Read1 : DataStoreRead  DataStoreName=Vin_Phase_B  IndexOptions=Index vector (dialog)  Indices=1  OutputSizes=1
  Function Caller1 : FunctionCaller  FunctionPrototype=SCI_A_Transmit(u)  InputArgumentSpecifications=<Enter example>  OutputArgumentSpecifications=<Enter example>
  Function Caller2 : FunctionCaller  FunctionPrototype=SCI_A_Transmit_Vin_Suffix()  InputArgumentSpecifications=<Enter example>  OutputArgumentSpecifications=<Enter example>
  Phase_B : Constant  Commented=on  Value=[66]  OutDataTypeStr=uint8
  SCI Transmit : c280xlib/SCI Transmit  Commented=on  sciModule=A  dataHead=''  dataTail=10  blockingMode=on  outputStatus=off
  wires:
  Data Store Read1/1 -> Function Caller1/1
  Phase_B/1 -> SCI Transmit/1

== system CLA_Sample/UART reporting @ 1Hz/Phase_B/Send Vin_rms (V) ==
  function : TriggerPort  TriggerType=function-call  VariantControl=(inherit)
  Data Store Read1 : DataStoreRead  DataStoreName=Vin_rms_Phase_B  IndexOptions=Index vector (dialog)  Indices=1  OutputSizes=1
  Function Caller1 : FunctionCaller  FunctionPrototype=SCI_A_Transmit(u)  InputArgumentSpecifications=<Enter example>  OutputArgumentSpecifications=<Enter example>
  Function Caller2 : FunctionCaller  FunctionPrototype=SCI_A_Transmit_Vin_rms_Suffix()  InputArgumentSpecifications=<Enter example>  OutputArgumentSpecifications=<Enter example>
  Phase_B : Constant  Commented=on  Value=[66]  OutDataTypeStr=uint8
  SCI Transmit : c280xlib/SCI Transmit  Commented=on  sciModule=A  dataHead=''  dataTail=10  blockingMode=on  outputStatus=off
  wires:
  Data Store Read1/1 -> Function Caller1/1
  Phase_B/1 -> SCI Transmit/1

== system CLA_Sample/UART reporting @ 1Hz/Phase_C/Duty_control_loop_Phase_C ==
  function : TriggerPort  TriggerType=function-call  VariantControl=(inherit)
  Data Store Read : DataStoreRead  Commented=on  DataStoreName=Vbulk_ADC_Average  IndexOptions=Index vector (dialog)  Indices=1  OutputSizes=1
  Data Store Read1 : DataStoreRead  DataStoreName=ePWM3A_CMPA_Phase_C  IndexOptions=Index vector (dialog)  Indices=1  OutputSizes=1
  Function Caller1 : FunctionCaller  FunctionPrototype=SCI_A_Transmit(u)  InputArgumentSpecifications=<Enter example>  OutputArgumentSpecifications=<Enter example>
  Function Caller2 : FunctionCaller  FunctionPrototype=SCI_A_Transmit_Polarity_Suffix()  InputArgumentSpecifications=<Enter example>  OutputArgumentSpecifications=<Enter example>
  Gain1 : Gain  Commented=on  Gain=DAC_Gain
  Gain7 : Gain  Commented=on  Gain=Vbulk_Divider_Gain
  Phase_C : Constant  Commented=on  Value=[67]  OutDataTypeStr=uint8
  SCI Transmit : c280xlib/SCI Transmit  Commented=on  sciModule=A  dataHead=''  dataTail=10  blockingMode=on  outputStatus=off
  wires:
  Data Store Read/1 -> Gain1/1
  Gain1/1 -> Gain7/1
  Data Store Read1/1 -> Function Caller1/1
  Phase_C/1 -> SCI Transmit/1

== system CLA_Sample/UART reporting @ 1Hz/Phase_C/Send Inductor_Current (A) ==
  function : TriggerPort  TriggerType=function-call  VariantControl=(inherit)
  Data Store Read : DataStoreRead  DataStoreName=Iin_rms_Phase_C  IndexOptions=Index vector (dialog)  Indices=1  OutputSizes=1
  Function Caller1 : FunctionCaller  FunctionPrototype=SCI_A_Transmit(u)  InputArgumentSpecifications=<Enter example>  OutputArgumentSpecifications=<Enter example>
  Function Caller2 : FunctionCaller  FunctionPrototype=SCI_A_Transmit_Current_Suffix()  InputArgumentSpecifications=<Enter example>  OutputArgumentSpecifications=<Enter example>
  Phase_C : Constant  Commented=on  Value=[67]  OutDataTypeStr=uint8
  SCI Transmit : c280xlib/SCI Transmit  Commented=on  sciModule=A  dataHead=''  dataTail=10  blockingMode=on  outputStatus=off
  wires:
  Data Store Read/1 -> Function Caller1/1
  Phase_C/1 -> SCI Transmit/1

== system CLA_Sample/UART reporting @ 1Hz/Phase_C/Send PFC_en_Phase_C ==
  function : TriggerPort  TriggerType=function-call  VariantControl=(inherit)
  Data Store Read : DataStoreRead  DataStoreName=PFC_en_Phase_C  IndexOptions=Index vector (dialog)  Indices=1  OutputSizes=1
  Function Caller1 : FunctionCaller  FunctionPrototype=SCI_A_Transmit(u)  InputArgumentSpecifications=<Enter example>  OutputArgumentSpecifications=<Enter example>
  Function Caller2 : FunctionCaller  FunctionPrototype=SCI_A_Transmit_Vp_Suffix()  InputArgumentSpecifications=<Enter example>  OutputArgumentSpecifications=<Enter example>
  Phase_C : Constant  Commented=on  Value=[67]  OutDataTypeStr=uint8
  SCI Transmit : c280xlib/SCI Transmit  Commented=on  sciModule=A  dataHead=''  dataTail=10  blockingMode=on  outputStatus=off
  wires:
  Data Store Read/1 -> Function Caller1/1
  Phase_C/1 -> SCI Transmit/1

== system CLA_Sample/UART reporting @ 1Hz/Phase_C/Send Vin (V) ==
  function : TriggerPort  TriggerType=function-call  VariantControl=(inherit)
  Data Store Read1 : DataStoreRead  DataStoreName=Vin_Phase_C  IndexOptions=Index vector (dialog)  Indices=1  OutputSizes=1
  Function Caller1 : FunctionCaller  FunctionPrototype=SCI_A_Transmit(u)  InputArgumentSpecifications=<Enter example>  OutputArgumentSpecifications=<Enter example>
  Function Caller2 : FunctionCaller  FunctionPrototype=SCI_A_Transmit_Vin_Suffix()  InputArgumentSpecifications=<Enter example>  OutputArgumentSpecifications=<Enter example>
  Phase_C : Constant  Commented=on  Value=[67]  OutDataTypeStr=uint8
  SCI Transmit : c280xlib/SCI Transmit  Commented=on  sciModule=A  dataHead=''  dataTail=10  blockingMode=on  outputStatus=off
  wires:
  Data Store Read1/1 -> Function Caller1/1
  Phase_C/1 -> SCI Transmit/1

== system CLA_Sample/UART reporting @ 1Hz/Phase_C/Send Vin_rms (V) ==
  function : TriggerPort  TriggerType=function-call  VariantControl=(inherit)
  Data Store Read1 : DataStoreRead  DataStoreName=Vin_rms_Phase_C  IndexOptions=Index vector (dialog)  Indices=1  OutputSizes=1
  Function Caller1 : FunctionCaller  FunctionPrototype=SCI_A_Transmit(u)  InputArgumentSpecifications=<Enter example>  OutputArgumentSpecifications=<Enter example>
  Function Caller2 : FunctionCaller  FunctionPrototype=SCI_A_Transmit_Vin_rms_Suffix()  InputArgumentSpecifications=<Enter example>  OutputArgumentSpecifications=<Enter example>
  Phase_C : Constant  Commented=on  Value=[67]  OutDataTypeStr=uint8
  SCI Transmit : c280xlib/SCI Transmit  Commented=on  sciModule=A  dataHead=''  dataTail=10  blockingMode=on  outputStatus=off
  wires:
  Data Store Read1/1 -> Function Caller1/1
  Phase_C/1 -> SCI Transmit/1

== system CLA_Sample/Calibration,RMS, Fault Protection @5kHz/Calibration/If Action Subsystem/If Action Subsystem ==
  In1 : Inport
  In2 : Inport  Port=2
  Action Port : ActionPort
  Constant : Constant  OutDataTypeStr=double
  Data Store Write1 : DataStoreWrite  DataStoreName=Calibration_Done_Phase_A  IndexOptions=Index vector (dialog)  Indices=1  OutputSizes=1
  Out1 : Outport
  Out2 : Outport  Port=2
  wires:
  In1/1 -> Out1/1
  Constant/1 -> Data Store Write1/1
  In2/1 -> Out2/1

== system CLA_Sample/Calibration,RMS, Fault Protection @5kHz/Fault checking/If Action Subsystem/Fault Check (Bulk UVP) ==
  function : TriggerPort  TriggerType=function-call  VariantControl=(inherit)
  Chart : Stateflow chart  TreatAsAtomicUnit=on
  Data Store Read1 : DataStoreRead  DataStoreName=Vbulk_ADC_Average  IndexOptions=Index vector (dialog)  Indices=1  OutputSizes=1
  Data Store Read2 : DataStoreRead  DataStoreName=Vbulk_Ref_ADC  IndexOptions=Index vector (dialog)  Indices=1  OutputSizes=1
  Data Store Read3 : DataStoreRead  DataStoreName=Soft_Start  IndexOptions=Index vector (dialog)  Indices=1  OutputSizes=1
  Data Store Read4 : DataStoreRead  DataStoreName=Vbulk_ADC  IndexOptions=Index vector (dialog)  Indices=1  OutputSizes=1
  Data Store Write : DataStoreWrite  DataStoreName=One_Shot_Bar  IndexOptions=Index vector (dialog)  Indices=1  OutputSizes=1
  Gain2 : Gain  Gain=DAC_Gain
  Gain3 : Gain  Gain=Vbulk_Divider_Gain  OutDataTypeStr=double
  wires:
  Data Store Read3/1 -> Chart/1(Soft_Start)
  Chart/1(Vbulk_UVP_Flag) -> Data Store Write/1
  Gain2/1 -> Gain3/1
  Data Store Read1/1 -> Gain2/1
  Gain3/1 -> Chart/4(Vbulk)
  Data Store Read2/1 -> Chart/3(Vbulk_Ref_ADC)
  Data Store Read4/1 -> Chart/2(Vbulk_ADC)

== system CLA_Sample/Calibration,RMS, Fault Protection @5kHz/Fault checking/If Action Subsystem/Output Voltage_Latch_OVP ==
  note: Output Voltage_Latch_OVP
  note: Vbulk_OVP_Threshold initialized in Data Store Memory
  function : TriggerPort  TriggerType=function-call  VariantControl=(inherit)
  Chart2 : Stateflow chart  TreatAsAtomicUnit=on
  Data Store Read : DataStoreRead  DataStoreName=Vbulk_ADC_Average  IndexOptions=Index vector (dialog)  Indices=1  OutputSizes=1
  Data Store Read1 : DataStoreRead  DataStoreName=Vbulk_OVP_Threshold  IndexOptions=Index vector (dialog)  Indices=1  OutputSizes=1
  Data Store Write1 : DataStoreWrite  DataStoreName=One_Shot_Bar  IndexOptions=Index vector (dialog)  Indices=1  OutputSizes=1
  Gain2 : Gain  Gain=DAC_Gain
  Gain3 : Gain  Gain=Vbulk_Divider_Gain  OutDataTypeStr=double
  wires:
  Chart2/1(One_Shot_Bar) -> Data Store Write1/1
  Data Store Read1/1 -> Chart2/2(Vbulk_OVP_Threshold)
  Gain2/1 -> Gain3/1
  Data Store Read/1 -> Gain2/1
  Gain3/1 -> Chart2/1(input_Vbulk)

== system CLA_Sample/Calibration,RMS, Fault Protection @5kHz/Fault checking/If Action Subsystem/PFC_en_update_3Phase ==
  function : TriggerPort  TriggerType=function-call  VariantControl=(inherit)
  Chart : Stateflow chart  TreatAsAtomicUnit=on
  Constant : Constant
  Data Store Read1 : DataStoreRead  DataStoreName=PFC_en_Phase_A  IndexOptions=Index vector (dialog)  Indices=1  OutputSizes=1
  Data Store Read2 : DataStoreRead  DataStoreName=PFC_en_Phase_B  IndexOptions=Index vector (dialog)  Indices=1  OutputSizes=1
  Data Store Read4 : DataStoreRead  DataStoreName=PFC_en_Phase_C  IndexOptions=Index vector (dialog)  Indices=1  OutputSizes=1
  Data Store Write : DataStoreWrite  DataStoreName=PFC_en  IndexOptions=Index vector (dialog)  Indices=1  OutputSizes=1
  wires:
  Chart/1(PFC_en) -> Data Store Write/1
  Data Store Read1/1 -> Chart/1(PFC_en_Phase_A)
  Constant/1 -> Chart/3(PFC_en_Phase_C), Chart/2(PFC_en_Phase_B)

== system CLA_Sample/Calibration,RMS, Fault Protection @5kHz/Fault checking/If Action Subsystem/PFC_en_update_Phase_A ==
  function : TriggerPort  TriggerType=function-call  VariantControl=(inherit)
  Chart : Stateflow chart  TreatAsAtomicUnit=on
  Data Store Read1 : DataStoreRead  DataStoreName=Vin_UVP_Flag_Phase_A  IndexOptions=Index vector (dialog)  Indices=1  OutputSizes=1
  Data Store Read2 : DataStoreRead  DataStoreName=Vin_OVP_Flag_Phase_A  IndexOptions=Index vector (dialog)  Indices=1  OutputSizes=1
  Data Store Read4 : DataStoreRead  DataStoreName=Iin_OCP_Flag_phase_A  IndexOptions=Index vector (dialog)  Indices=1  OutputSizes=1
  Data Store Write : DataStoreWrite  DataStoreName=PFC_en_Phase_A  IndexOptions=Index vector (dialog)  Indices=1  OutputSizes=1
  Data Store Write1 : DataStoreWrite  DataStoreName=PFC_en1  IndexOptions=Index vector (dialog)  Indices=1  OutputSizes=1
  wires:
  Chart/2(PFC_en1) -> Data Store Write1/1
  Data Store Read1/1 -> Chart/1(Vin_UVP_Flag)
  Data Store Read2/1 -> Chart/2(Vin_OVP_Flag)
  Chart/1(PFC_en) -> Data Store Write/1
  Data Store Read4/1 -> Chart/3(Iin_OCP_Flag)

== system CLA_Sample/Calibration,RMS, Fault Protection @5kHz/Fault checking/If Action Subsystem/PFC_en_update_Phase_B ==
  function : TriggerPort  TriggerType=function-call  VariantControl=(inherit)
  Chart : Stateflow chart  TreatAsAtomicUnit=on
  Data Store Read : DataStoreRead  Commented=on  DataStoreName=counter_Relay  IndexOptions=Index vector (dialog)  Indices=1  OutputSizes=1
  Data Store Read1 : DataStoreRead  DataStoreName=Vin_UVP_Flag_Phase_B  IndexOptions=Index vector (dialog)  Indices=1  OutputSizes=1
  Data Store Read2 : DataStoreRead  DataStoreName=Vin_OVP_Flag_Phase_B  IndexOptions=Index vector (dialog)  Indices=1  OutputSizes=1
  Data Store Read4 : DataStoreRead  DataStoreName=Iin_OCP_Flag_phase_B  IndexOptions=Index vector (dialog)  Indices=1  OutputSizes=1
  Data Store Write : DataStoreWrite  DataStoreName=PFC_en_Phase_B  IndexOptions=Index vector (dialog)  Indices=1  OutputSizes=1
  Data Store Write1 : DataStoreWrite  DataStoreName=PFC_en1  IndexOptions=Index vector (dialog)  Indices=1  OutputSizes=1
  Data Store Write2 : DataStoreWrite  Commented=on  DataStoreName=counter_Relay  IndexOptions=Index vector (dialog)  Indices=1  OutputSizes=1
  Product : Product  Commented=on
  wires:
  Chart/2(PFC_en1) -> Data Store Write1/1
  Data Store Read1/1 -> Chart/1(Vin_UVP_Flag)
  Data Store Read/1 -> Product/2
  Product/1 -> Data Store Write2/1
  Chart/1(PFC_en) -> Product/1, Data Store Write/1
  Data Store Read2/1 -> Chart/2(Vin_OVP_Flag)
  Data Store Read4/1 -> Chart/3(Iin_OCP_Flag)
